simulink model "Task_3"  (R2023b)
settings: Solver=FixedStepAuto  StartTime=0.0  StopTime=tfinal  FixedStep=dt  RelTol=1e-3
values from neighbouring files (symbols this model uses):
  F_gravity_0 = mass*gravity*[sin(states_0(8)) ... (first row only)    [Data_edit.m]
  gravity = Airplane_data(52)    [Data_edit.m]
  Ixx = Airplane_data(53)    [Data_edit.m]
  Iyy = Airplane_data(54)    [Data_edit.m]
  Izz = Airplane_data(55)    [Data_edit.m]
  M0 = [0;0;0]    [Data_edit.m]
  mass = Airplane_data(51)    [Data_edit.m]
  Matrix_controls = [ 0             Xde             Xdth            0 ... (first row only)    [Data_edit.m]
  Matrix_states = [Xu   0   Xw  0   0   0   0 ... (first row only)    [Data_edit.m]
  saifStruct = struct()    [Struct.m]
  states_0 = Airplane_data(4:15)    [Data_edit.m]
libraries: simulink_extras x9, shared6dof x1, aerolibasang x1, dspsigops x1
settings Model: Creator=Saif Mohamed  LastModifiedBy=Saif Mohamed

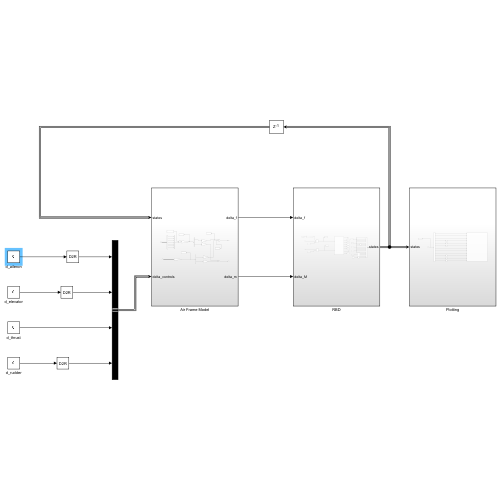
[thumbnail: Simulink's stored preview of the top-level diagram]
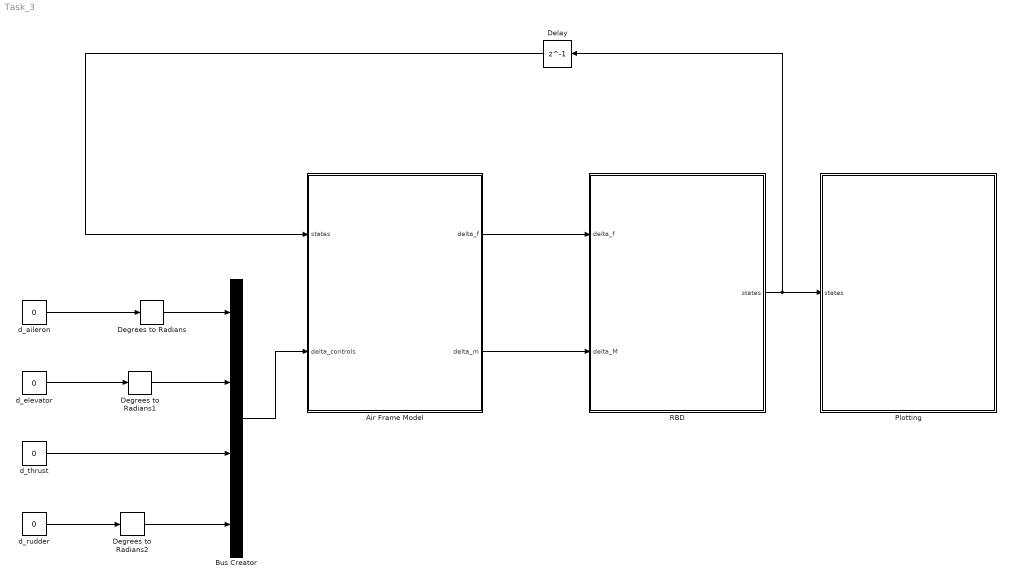
== system Task_3 ==
  Air Frame Model : Subsystem
  Bus Creator : BusCreator  Inputs=4
  Degrees to Radians : simulink_extras/Transformations/Degrees to Radians
  Degrees to Radians1 : simulink_extras/Transformations/Degrees to Radians
  Degrees to Radians2 : simulink_extras/Transformations/Degrees to Radians
  Delay : Delay  DelayLength=1  InitialCondition=saifStruct
  Plotting : Subsystem
  RBD : Subsystem
  d_aileron : Constant  Value=0
  d_elevator : Constant  Value=0
  d_rudder : Constant  Value=0
  d_thrust : Constant  Value=0
  wires:
  RBD/1(states) -> Delay/1, Plotting/1(states)
  Air Frame Model/1(delta_f) -> RBD/1(delta_f)
  Air Frame Model/2(delta_m) -> RBD/2(delta_M)
  d_elevator/1 -> Degrees to Radians1/1
  d_aileron/1 -> Degrees to Radians/1
  d_rudder/1 -> Degrees to Radians2/1
  d_thrust/1 -> Bus Creator/3
  Bus Creator/1 -> Air Frame Model/2(delta_controls)
  Degrees to Radians/1 -> Bus Creator/1
  Degrees to Radians1/1 -> Bus Creator/2
  Degrees to Radians2/1 -> Bus Creator/4
  Delay/1 -> Air Frame Model/1(states)

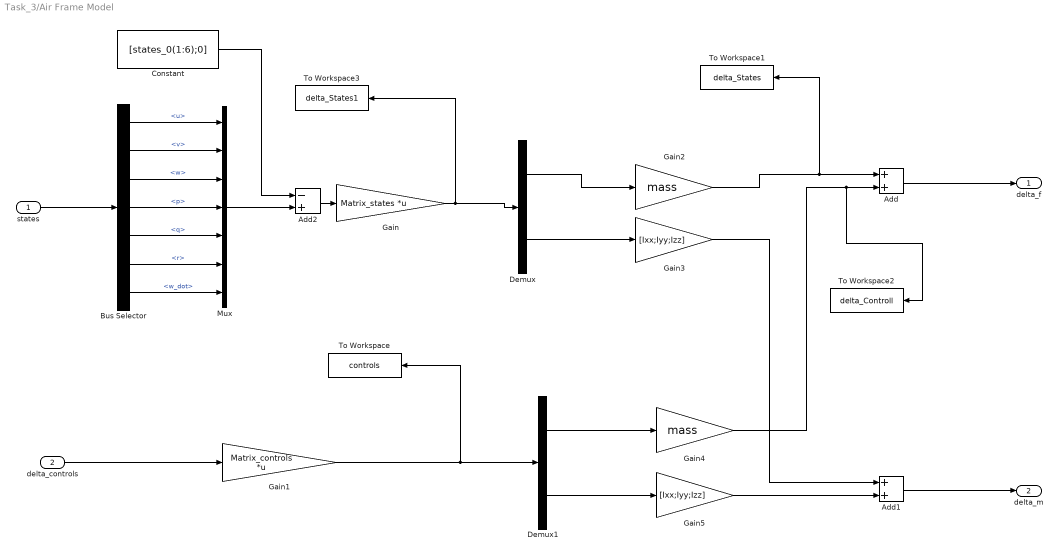
== system Task_3/Air Frame Model ==
  states : Inport
  delta_controls : Inport  Port=2
  Add : Sum
  Add1 : Sum
  Add2 : Sum  Inputs=-+
  Bus Selector : BusSelector  OutputSignals=u,v,w,p,q,r,w_dot
  Constant : Constant  Value=[states_0(1:6);0]
  Demux : Demux  Outputs=2
  Demux1 : Demux  Outputs=2
  Gain : Gain  Gain=Matrix_states  Multiplication=Matrix(K*u)
  Gain1 : Gain  Gain=Matrix_controls  Multiplication=Matrix(K*u)
  Gain2 : Gain  Gain=mass
  Gain3 : Gain  Gain=[Ixx;Iyy;Izz]
  Gain4 : Gain  Gain=mass
  Gain5 : Gain  Gain=[Ixx;Iyy;Izz]
  Mux : Mux  Inputs=7
  To Workspace : ToWorkspace  VariableName=controls  SampleTime=-1
  To Workspace1 : ToWorkspace  VariableName=delta_States  SampleTime=-1
  To Workspace2 : ToWorkspace  VariableName=delta_Controll  SampleTime=-1
  To Workspace3 : ToWorkspace  VariableName=delta_States1  SampleTime=-1
  delta_f : Outport
  delta_m : Outport  Port=2
  wires:
  Gain/1 -> To Workspace3/1, Demux/1
  Demux/1 -> Gain2/1
  Demux/2 -> Gain3/1
  Demux1/2 -> Gain5/1
  Demux1/1 -> Gain4/1
  Gain1/1 -> To Workspace/1, Demux1/1
  Gain2/1 -> To Workspace1/1, Add/1
  Gain4/1 -> To Workspace2/1, Add/2
  Gain5/1 -> Add1/2
  Gain3/1 -> Add1/1
  Add/1 -> delta_f/1
  Add1/1 -> delta_m/1
  states/1 -> Bus Selector/1
  Bus Selector/1 -> Mux/1  "<u>"
  Bus Selector/2 -> Mux/2  "<v>"
  Bus Selector/3 -> Mux/3  "<w>"
  Bus Selector/4 -> Mux/4  "<p>"
  Bus Selector/5 -> Mux/5  "<q>"
  Bus Selector/6 -> Mux/6  "<r>"
  Bus Selector/7 -> Mux/7  "<w_dot>"
  Add2/1 -> Gain/1
  Mux/1 -> Add2/2
  Constant/1 -> Add2/1
  delta_controls/1 -> Gain1/1

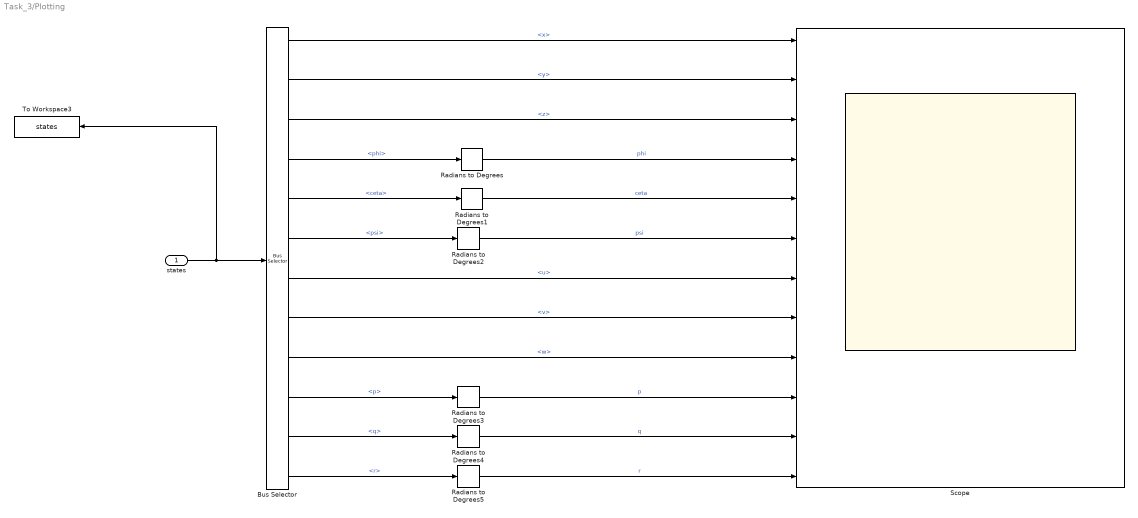
== system Task_3/Plotting ==
  states : Inport
  Bus Selector : BusSelector  OutputSignals=x,y,z,phi,ceta,psi,u,v,w,p,q,r
  Radians to Degrees{,1..5} (6 alike) : simulink_extras/Transformations/Radians to Degrees
  Scope : Scope  NumInputPorts=12
  To Workspace3 : ToWorkspace  VariableName=states  SampleTime=-1
  wires:
  states/1 -> To Workspace3/1, Bus Selector/1
  Bus Selector/1 -> Scope/1  "<x>"
  Bus Selector/2 -> Scope/2  "<y>"
  Bus Selector/3 -> Scope/3  "<z>"
  Bus Selector/4 -> Radians to Degrees/1  "<phi>"
  Bus Selector/5 -> Radians to Degrees1/1  "<ceta>"
  Bus Selector/6 -> Radians to Degrees2/1  "<psi>"
  Bus Selector/7 -> Scope/7  "<u>"
  Bus Selector/8 -> Scope/8  "<v>"
  Bus Selector/9 -> Scope/9  "<w>"
  Bus Selector/10 -> Radians to Degrees3/1  "<p>"
  Bus Selector/11 -> Radians to Degrees4/1  "<q>"
  Bus Selector/12 -> Radians to Degrees5/1  "<r>"
  Radians to Degrees/1 -> Scope/4  "phi"
  Radians to Degrees1/1 -> Scope/5  "ceta"
  Radians to Degrees2/1 -> Scope/6  "psi"
  Radians to Degrees3/1 -> Scope/10  "p"
  Radians to Degrees4/1 -> Scope/11  "q"
  Radians to Degrees5/1 -> Scope/12  "r"

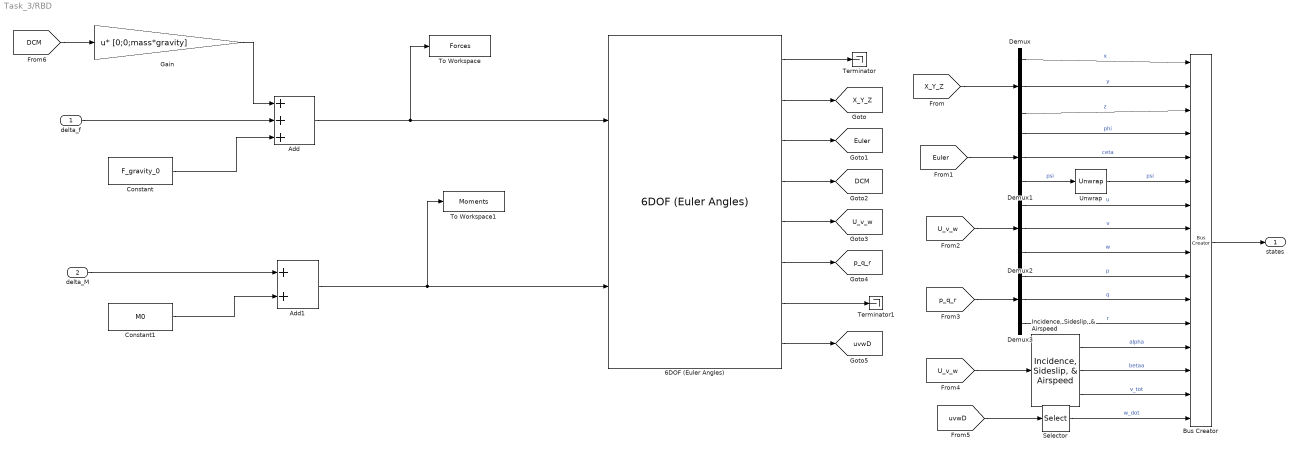
== system Task_3/RBD ==
  delta_f : Inport
  delta_M : Inport  Port=2
  6DOF (Euler Angles) : shared6dof/6DOF (Euler Angles)  units=English (Velocity in ft/s)  mtype=Fixed  rep=Euler Angles  xme_0=states_0(10:12)  Vm_0=states_0(1:3)  eul_0=states_0(7:9)  pm_0=states_0(4:6)  mass_0=mass  mass_e=0.5  mass_f=2.0  inertia=I  inertia_e=eye(3)  inertia_f=2*eye(3)  k_quat=1.0  vre_flag=on  abi_flag=off  aMode=0  xme_statename=''  Vm_statename=''  eul_statename=''  quat_statename=''  pm_statename=''  mass_statename=''
  Add : Sum  Inputs=+++
  Add1 : Sum
  Bus Creator : BusCreator  Inputs=16
  Constant : Constant  Value=F_gravity_0
  Constant1 : Constant  Value=M0
  Demux{,1..3} (4 alike) : Demux  Outputs=3
  Gain : Gain  Gain=[0;0;mass*gravity]  Multiplication=Matrix(u*K)
  "Incidence, Sideslip, & Airspeed" : aerolibasang/Incidence, Sideslip, & Airspeed
  Selector : Selector  InputPortWidth=3  IndexOptions=Index vector (dialog)  Indices=[3]  OutputSizes=1
  Terminator : Terminator
  Terminator1 : Terminator
  To Workspace : ToWorkspace  VariableName=Forces  SampleTime=-1
  To Workspace1 : ToWorkspace  VariableName=Moments  SampleTime=-1
  Unwrap : dspsigops/Unwrap  tol=pi  InputProcessing=Columns as channels (frame based)  running=off
  states : Outport
  tag scope: DCM=global, Euler=global, U_v_w=global, X_Y_Z=global, p_q_r=global, uvwD=global
  wires:
  6DOF (Euler Angles)/1 -> Terminator/1
  6DOF (Euler Angles)/2 -> [X_Y_Z]
  6DOF (Euler Angles)/3 -> [Euler]
  6DOF (Euler Angles)/4 -> [DCM]
  6DOF (Euler Angles)/5 -> [U_v_w]
  6DOF (Euler Angles)/6 -> [p_q_r]
  6DOF (Euler Angles)/7 -> Terminator1/1
  6DOF (Euler Angles)/8 -> [uvwD]
  [X_Y_Z] -> Demux/1
  [Euler] -> Demux1/1
  [U_v_w] -> Demux2/1
  [p_q_r] -> Demux3/1
  Demux/1 -> Bus Creator/1  "x"
  Demux/2 -> Bus Creator/2  "y"
  Demux/3 -> Bus Creator/3  "z"
  Demux1/1 -> Bus Creator/4  "phi"
  Demux1/2 -> Bus Creator/5  "ceta"
  Demux1/3 -> Unwrap/1  "psi"
  Demux2/1 -> Bus Creator/7  "u"
  Demux2/2 -> Bus Creator/8  "v"
  Demux2/3 -> Bus Creator/9  "w"
  Demux3/1 -> Bus Creator/10  "p"
  Demux3/2 -> Bus Creator/11  "q"
  Demux3/3 -> Bus Creator/12  "r"
  [U_v_w] -> "Incidence, Sideslip, & Airspeed"/1
  "Incidence, Sideslip, & Airspeed"/2 -> Bus Creator/14  "betaa"
  "Incidence, Sideslip, & Airspeed"/1 -> Bus Creator/13  "alpha"
  "Incidence, Sideslip, & Airspeed"/3 -> Bus Creator/15  "v_tot"
  [uvwD] -> Selector/1
  Selector/1 -> Bus Creator/16  "w_dot"
  Bus Creator/1 -> states/1
  delta_f/1 -> Add/2
  [DCM] -> Gain/1
  Gain/1 -> Add/1
  Constant/1 -> Add/3
  delta_M/1 -> Add1/1
  Constant1/1 -> Add1/2
  Add1/1 -> To Workspace1/1, 6DOF (Euler Angles)/2
  Unwrap/1 -> Bus Creator/6  "psi"
  Add/1 -> To Workspace/1, 6DOF (Euler Angles)/1
